simulink model "SamplePendulum"  (R2020b)
settings: Solver=ode45  StartTime=0.0  StopTime=inf  FixedStep=0.001  RelTol=1e-5  AbsTol=1e-6
model workspace (MAT data in the model file):
  I = 0
  c = 0
  g = 9.81
  l = 1
  m = 1
  max_tau = 2
  theta0 = 0
  theta_dot0 = 0
undefined symbols (not defined in the file): f
libraries: instrumentlib x3
settings Model: ParameterArgumentNames=theta0,theta_dot0  OrderedModelArguments=off  Creator=The MathWorks, Inc.  LastModifiedBy=Mark
settings SolverCC: AutoScaleAbsTol=off
settings DataIOCC: LimitDataPoints=on  SaveFormat=Array  SaveState=on
settings OptimizationCC: BlockReduction=off  BooleanDataType=off  LifeSpan=inf
settings DebuggingCC: SaveWithParameterizedLinksMsg=none  SignalResolutionControl=TryResolveAllWithWarning  SFUnexpectedBacktrackingDiag=warning  SFNoUnconditionalDefaultTransitionDiag=warning  SFExecutionAtInitializationDiag=none  ArithmeticOperatorsInVariantConditions=warning
settings HardwareCC: ProdBitPerPointer=32  ProdBitPerSizeT=32  ProdBitPerPtrDiffT=32  ProdLargestAtomicFloat=None  ProdIntDivRoundTo=Undefined  ProdEndianess=Unspecified  ProdWordSize=32  ProdHWDeviceType=32-bit Generic  TargetUnknown=on
settings ModelReferenceCC: PropagateSignalLabelsOutOfModel=off
settings SFSimCC: SimUseLocalCustomCode=off  CustomCodeUndefinedFunction=UseInterfaceOnly
settings RTWCC: RTWUseLocalCustomCode=off
settings CodeAppCC: StateflowObjectComments=on
settings GRTTargetCC: TargetLangStandard=C89/C90 (ANSI)
settings ConfigComp: CovMetricSettings=dw  CovSaveCumulativeToWorkspaceVar=on  CovSaveSingleToWorkspaceVar=on  CovExternalEMLEnable=off

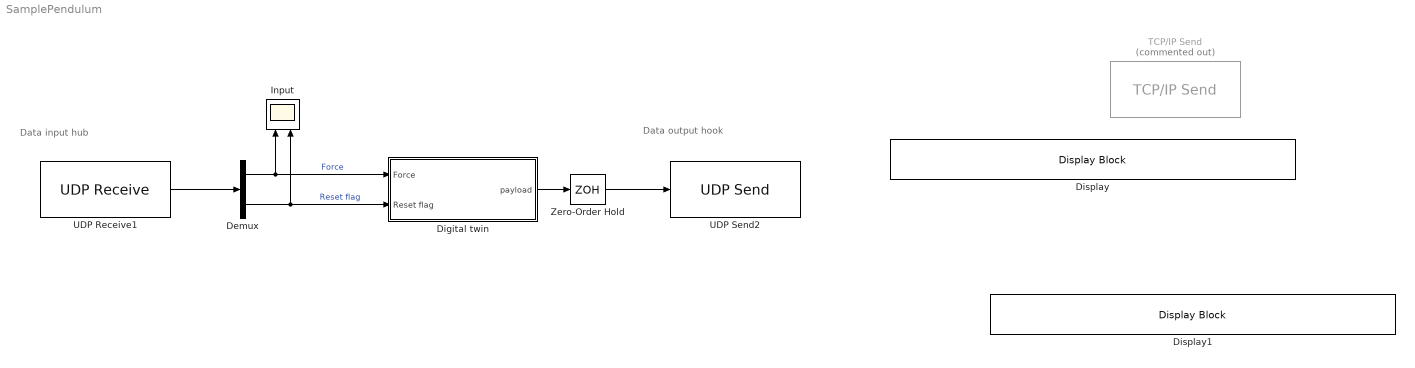
== system SamplePendulum ==
  note: Data output hook
  note: Data input hub
  Demux : Demux  Outputs=2
  Digital twin : Subsystem
  Display : DisplayBlock  LabelPosition=Hide  Format=short  Transparency=1
  Display1 : DisplayBlock  LabelPosition=Hide  Format=short  Transparency=1
  Input : Scope  NumInputPorts=2
  TCP/IP Send : instrumentlib/TCP//IP Send  Commented=on  Host=127.0.0.1  Port=16385  EnableBlockingMode=on  Timeout=60  ByteOrder=BigEndian  TransferDelay=on
  UDP Receive1 : instrumentlib/UDP Receive  Host=localhost  Port=9090  LocalPort=16384  EnablePortSharing=off  GetLatestData=off  DataSize="[2  1]"  DataType=double  ASCIIFormatting=%f,  Terminator=LF  ByteOrder=BigEndian  EnableBlockingMode=on  Timeout=30  SampleTime=0.05  LocalAddress=0.0.0.0
  UDP Send2 : instrumentlib/UDP Send  Host=127.0.0.1  Port=16385  LocalPort=-1  EnablePortSharing=on  ByteOrder=BigEndian  OutputDatagramPacketSize=512  EnableBlockingMode=on  LocalAddress=0.0.0.0
  Zero-Order Hold : ZeroOrderHold  SampleTime=0.05
  wires:
  Demux/1 -> Input/1, Digital twin/1(Force)  "Force"
  Demux/2 -> Digital twin/2(Reset flag), Input/2  "Reset flag"
  UDP Receive1/1 -> Demux/1
  Zero-Order Hold/1 -> UDP Send2/1
  Digital twin/1(payload) -> Zero-Order Hold/1

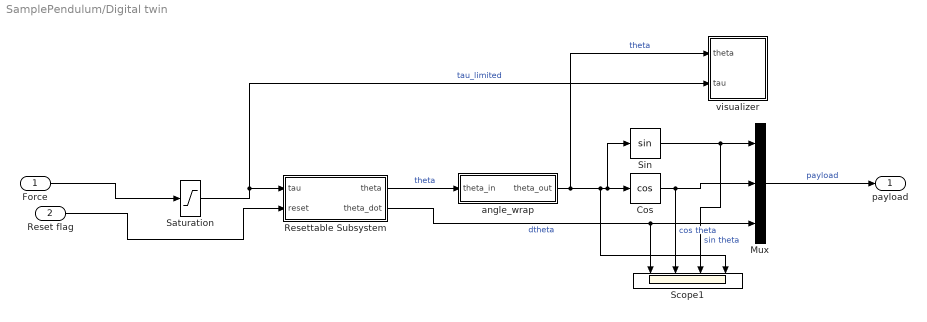
== system SamplePendulum/Digital twin ==
  Force : Inport
  Reset flag : Inport  Port=2
  Cos : Trigonometry  Operator=cos
  Mux : Mux  Inputs=3
  Resettable Subsystem : Subsystem  TreatAsAtomicUnit=on
  Saturation : Saturate  UpperLimit=2  LowerLimit=-2
  Scope1 : Scope  NumInputPorts=4
  Sin : Trigonometry
  angle_wrap : Subsystem
  visualizer : Subsystem
  payload : Outport
  wires:
  Resettable Subsystem/2(theta_dot) -> Mux/3, Scope1/1  "dtheta"
  Cos/1 -> Mux/2, Scope1/2  "cos theta"
  Mux/1 -> payload/1  "payload"
  Saturation/1 -> visualizer/2(tau), Resettable Subsystem/1(tau)  "tau_limited"
  Reset flag/1 -> Resettable Subsystem/2(reset)
  Resettable Subsystem/1(theta) -> angle_wrap/1(theta_in)  "theta"
  Sin/1 -> Mux/1, Scope1/3  "sin theta"
  Force/1 -> Saturation/1
  angle_wrap/1(theta_out) -> Scope1/4, Cos/1, Sin/1, visualizer/1(theta)  "theta"

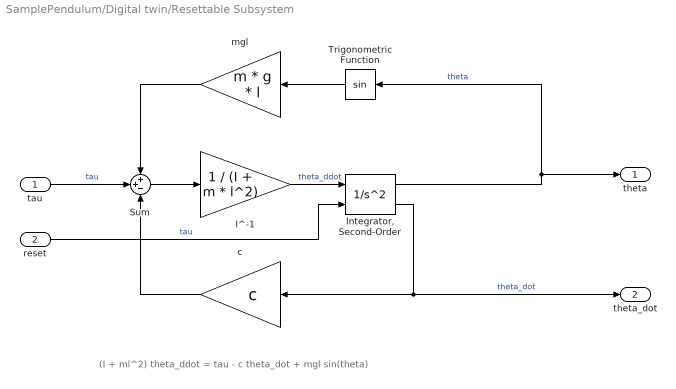
== system SamplePendulum/Digital twin/Resettable Subsystem ==
  note: (I + ml^2) theta_ddot = tau - c theta_dot + mgl sin(theta)
  tau : Inport
  reset : Inport  Port=2
  I^-1 : Gain  Gain=1 / (I + m * l^2)
  "Integrator, Second-Order" : SecondOrderIntegrator  ICX=pi  UpperLimitX=1  LowerLimitX=0  StateNameX='theta'  ICDXDT=0  StateNameDXDT='theta_dot'  ExternalReset=rising
  Sum : Sum  Inputs=++-
  Trigonometric Function : Trigonometry
  c : Gain  Gain=c
  mgl : Gain  Gain=m * g * l
  theta : Outport  VectorParamsAs1DForOutWhenUnconnected=off
  theta_dot : Outport  Port=2  VectorParamsAs1DForOutWhenUnconnected=off
  wires:
  tau/1 -> Sum/2  "tau"
  c/1 -> Sum/3
  Sum/1 -> I^-1/1
  "Integrator, Second-Order"/1 -> theta/1, Trigonometric Function/1  "theta"
  "Integrator, Second-Order"/2 -> c/1, theta_dot/1  "theta_dot"
  mgl/1 -> Sum/1
  Trigonometric Function/1 -> mgl/1
  I^-1/1 -> "Integrator, Second-Order"/1  "theta_ddot"
  reset/1 -> "Integrator, Second-Order"/2  "tau"

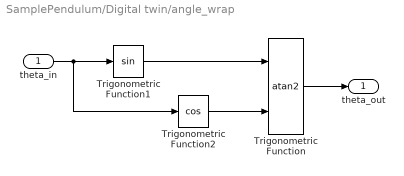
== system SamplePendulum/Digital twin/angle_wrap ==
  theta_in : Inport
  Trigonometric Function : Trigonometry  Operator=atan2
  Trigonometric Function1 : Trigonometry
  Trigonometric Function2 : Trigonometry  Operator=cos
  theta_out : Outport  VectorParamsAs1DForOutWhenUnconnected=off
  wires:
  theta_in/1 -> Trigonometric Function2/1, Trigonometric Function1/1
  Trigonometric Function/1 -> theta_out/1
  Trigonometric Function1/1 -> Trigonometric Function/1
  Trigonometric Function2/1 -> Trigonometric Function/2

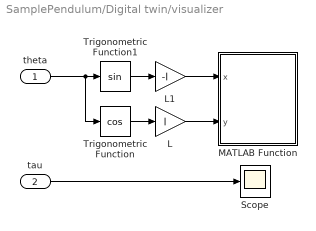
== system SamplePendulum/Digital twin/visualizer ==
  theta : Inport
  tau : Inport  Port=2
  L : Gain  Gain=l
  L1 : Gain  Gain=-l
  MATLAB Function : MATLAB Function  TreatAsAtomicUnit=on
  Scope : Scope
  Trigonometric Function : Trigonometry  Operator=cos
  Trigonometric Function1 : Trigonometry
  wires:
  theta/1 -> Trigonometric Function/1, Trigonometric Function1/1
  L1/1 -> MATLAB Function/1(x)
  Trigonometric Function/1 -> L/1
  L/1 -> MATLAB Function/2(y)
  Trigonometric Function1/1 -> L1/1
  tau/1 -> Scope/1

== matlab function SamplePendulum/Digital twin/visualizer/MATLAB Function ==
  settings: updateMethod=DISCRETE
  data: x input; y input
function plotPend(x,y)
% plot the simple pendulum
coder.extrinsic('rl.env.viz.plotSimplePendulum');
rl.env.viz.plotSimplePendulum(x,y);
